simulink model "BlankCntrlr_model2013b"  (Simulink 8.2)
settings: Solver=FixedStepDiscrete  StartTime=0.0  StopTime=inf  FixedStep=Ts  RelTol=1e-3
settings Model: Creator=NA  LastModifiedBy=jbutterw
settings DataIOCC: SaveOutput=off  SignalLogging=off  SaveTime=off
settings OptimizationCC: InlineParams=on
settings DebuggingCC: FcnCallInpInsideContextMsg=EnableAllAsWarning  FrameProcessingCompatibilityMsg=error
settings SFSimCC: SimParseCustomCode=off
settings RTWCC: SystemTargetFile=discon.tlc  GenCodeOnly=on  TemplateMakefile=discon.tmf  Description=DISCON DLL Target (for use with GH BLADED)  RTWCompilerOptimization=On
settings GRTTargetCC: CodeReplacementLibrary=C89/C90 (ANSI)  ExtModeMexFile=noextcomm

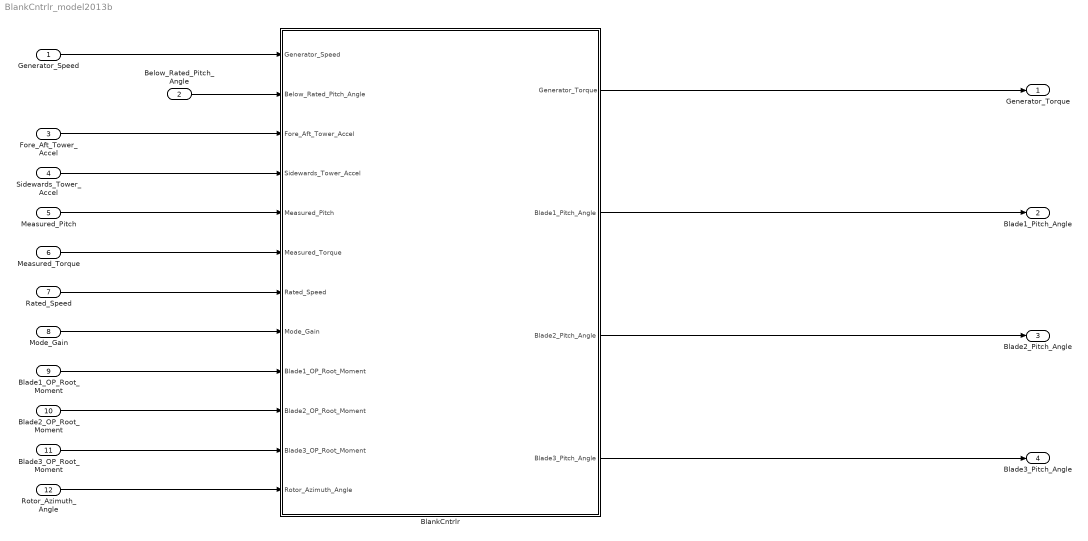
== system BlankCntrlr_model2013b ==
  Generator_Speed : Inport  PortDimensions=1
  Below_Rated_Pitch_Angle : Inport  Port=2  PortDimensions=1
  Fore_Aft_Tower_Accel : Inport  Port=3  PortDimensions=1
  Sidewards_Tower_Accel : Inport  Port=4  PortDimensions=1
  Measured_Pitch : Inport  Port=5  PortDimensions=1
  Measured_Torque : Inport  Port=6  PortDimensions=1
  Rated_Speed : Inport  Port=7  PortDimensions=1
  Mode_Gain : Inport  Port=8  PortDimensions=1
  Blade1_OP_Root_Moment : Inport  Port=9  PortDimensions=1
  Blade2_OP_Root_Moment : Inport  Port=10  PortDimensions=1
  Blade3_OP_Root_Moment : Inport  Port=11  PortDimensions=1
  Rotor_Azimuth_Angle : Inport  Port=12  PortDimensions=1
  BlankCntrlr : Subsystem  InitFcn=|
      | %LoadBUCkeyrootparams
      | %LoadBUCparams
      | %LoadBUCscript
  Generator_Torque : Outport  PortDimensions=1
  Blade1_Pitch_Angle : Outport  Port=2  PortDimensions=1
  Blade2_Pitch_Angle : Outport  Port=3  PortDimensions=1
  Blade3_Pitch_Angle : Outport  Port=4  PortDimensions=1
  wires:
  Generator_Speed/1 -> BlankCntrlr/1(Generator_Speed)
  Below_Rated_Pitch_Angle/1 -> BlankCntrlr/2(Below_Rated_Pitch_Angle)
  Fore_Aft_Tower_Accel/1 -> BlankCntrlr/3(Fore_Aft_Tower_Accel)
  Sidewards_Tower_Accel/1 -> BlankCntrlr/4(Sidewards_Tower_Accel)
  Measured_Pitch/1 -> BlankCntrlr/5(Measured_Pitch)
  Measured_Torque/1 -> BlankCntrlr/6(Measured_Torque)
  Rated_Speed/1 -> BlankCntrlr/7(Rated_Speed)
  Mode_Gain/1 -> BlankCntrlr/8(Mode_Gain)
  Blade1_OP_Root_Moment/1 -> BlankCntrlr/9(Blade1_OP_Root_Moment)
  Blade2_OP_Root_Moment/1 -> BlankCntrlr/10(Blade2_OP_Root_Moment)
  Blade3_OP_Root_Moment/1 -> BlankCntrlr/11(Blade3_OP_Root_Moment)
  Rotor_Azimuth_Angle/1 -> BlankCntrlr/12(Rotor_Azimuth_Angle)
  BlankCntrlr/1(Generator_Torque) -> Generator_Torque/1
  BlankCntrlr/2(Blade1_Pitch_Angle) -> Blade1_Pitch_Angle/1
  BlankCntrlr/3(Blade2_Pitch_Angle) -> Blade2_Pitch_Angle/1
  BlankCntrlr/4(Blade3_Pitch_Angle) -> Blade3_Pitch_Angle/1

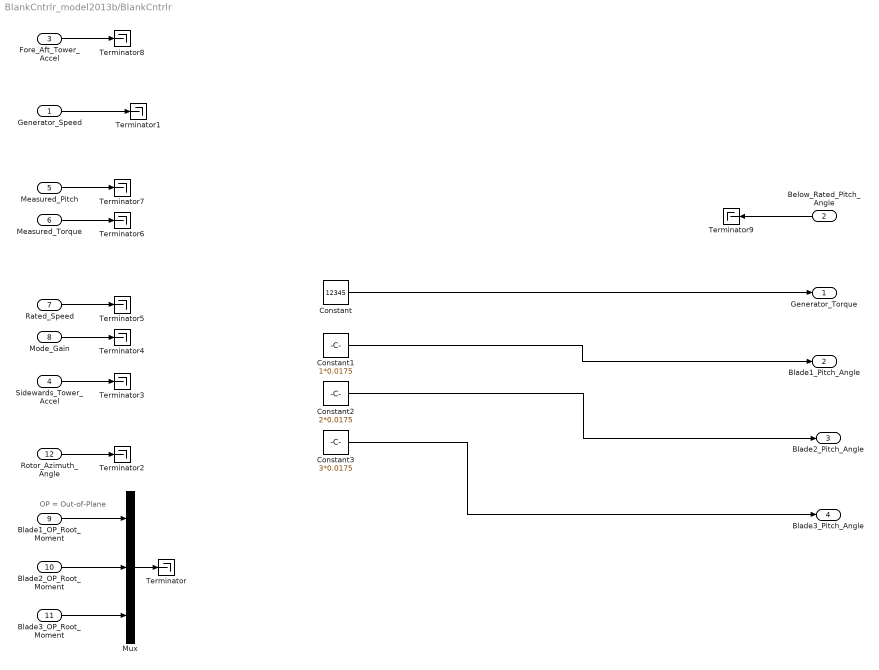
== system BlankCntrlr_model2013b/BlankCntrlr ==
  note: OP = Out-of-Plane
  Generator_Speed : Inport  PortDimensions=1
  Below_Rated_Pitch_Angle : Inport  Port=2  PortDimensions=1
  Fore_Aft_Tower_Accel : Inport  Port=3  PortDimensions=1
  Sidewards_Tower_Accel : Inport  Port=4  PortDimensions=1
  Measured_Pitch : Inport  Port=5  PortDimensions=1
  Measured_Torque : Inport  Port=6  PortDimensions=1
  Rated_Speed : Inport  Port=7  PortDimensions=1
  Mode_Gain : Inport  Port=8  PortDimensions=1
  Blade1_OP_Root_Moment : Inport  Port=9  PortDimensions=1
  Blade2_OP_Root_Moment : Inport  Port=10  PortDimensions=1
  Blade3_OP_Root_Moment : Inport  Port=11  PortDimensions=1
  Rotor_Azimuth_Angle : Inport  Port=12  PortDimensions=1
  Constant : Constant  Value=12345
  Constant1 : Constant  Value=1*0.0175
  Constant2 : Constant  Value=2*0.0175
  Constant3 : Constant  Value=3*0.0175
  Mux : Mux  Inputs=3
  Terminator{,1..9} (10 alike) : Terminator
  Generator_Torque : Outport  PortDimensions=1
  Blade1_Pitch_Angle : Outport  Port=2  PortDimensions=1
  Blade2_Pitch_Angle : Outport  Port=3  PortDimensions=1
  Blade3_Pitch_Angle : Outport  Port=4  PortDimensions=1
  wires:
  Blade2_OP_Root_Moment/1 -> Mux/2
  Blade3_OP_Root_Moment/1 -> Mux/3
  Rotor_Azimuth_Angle/1 -> Terminator2/1
  Measured_Torque/1 -> Terminator6/1
  Fore_Aft_Tower_Accel/1 -> Terminator8/1
  Sidewards_Tower_Accel/1 -> Terminator3/1
  Blade1_OP_Root_Moment/1 -> Mux/1
  Rated_Speed/1 -> Terminator5/1
  Mode_Gain/1 -> Terminator4/1
  Mux/1 -> Terminator/1
  Measured_Pitch/1 -> Terminator7/1
  Generator_Speed/1 -> Terminator1/1
  Constant/1 -> Generator_Torque/1
  Below_Rated_Pitch_Angle/1 -> Terminator9/1
  Constant1/1 -> Blade1_Pitch_Angle/1
  Constant2/1 -> Blade2_Pitch_Angle/1
  Constant3/1 -> Blade3_Pitch_Angle/1
